simulink model "prob4_214869"  (R2020a)
settings: Solver=VariableStepAuto  StartTime=0.0  StopTime=10.0  RelTol=1e-3
settings Model: Creator=sonal  LastModifiedBy=sonal

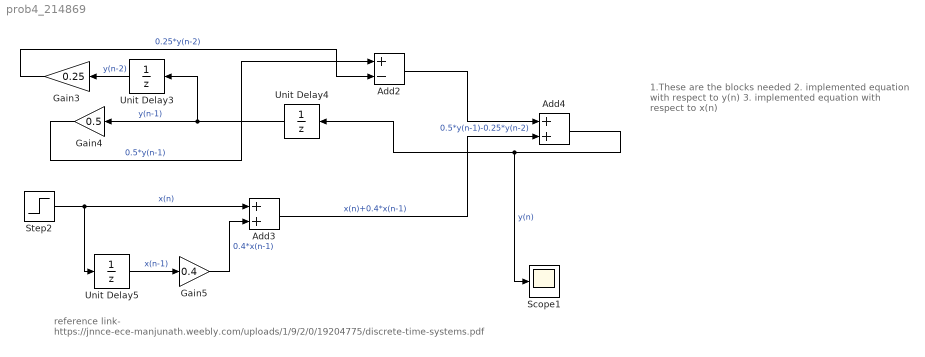
== system prob4_214869 ==
  note: reference link- https://jnnce-ece-manjunath.weebly.com/uploads/1/9/2/0/19204775/discrete-time-systems.pdf
  note: 1.These are the blocks needed
      | 2. implemented equation with respect to y(n)
      | 3. implemented equation with respect to x(n)
  Add2 : Sum  Inputs=+-
  Add3 : Sum
  Add4 : Sum
  Gain3 : Gain  Gain=0.25
  Gain4 : Gain  Gain=0.5
  Gain5 : Gain  Gain=0.4
  Scope1 : Scope
  Step2 : Step  SampleTime=0.01
  Unit Delay3 : UnitDelay  SampleTime=-1  HasFrameUpgradeWarning=on
  Unit Delay4 : UnitDelay  SampleTime=-1  HasFrameUpgradeWarning=on
  Unit Delay5 : UnitDelay  SampleTime=-1  HasFrameUpgradeWarning=on
  wires:
  Gain4/1 -> Add2/1  "0.5*y(n-1)"
  Gain3/1 -> Add2/2  "0.25*y(n-2)"
  Add4/1 -> Scope1/1, Unit Delay4/1  "y(n)"
  Unit Delay4/1 -> Unit Delay3/1, Gain4/1  "y(n-1)"
  Unit Delay3/1 -> Gain3/1  "y(n-2)"
  Step2/1 -> Unit Delay5/1, Add3/1  "x(n)"
  Gain5/1 -> Add3/2  "0.4*x(n-1)"
  Add3/1 -> Add4/2  "x(n)+0.4*x(n-1)"
  Unit Delay5/1 -> Gain5/1  "x(n-1)"
  Add2/1 -> Add4/1  "0.5*y(n-1)-0.25*y(n-2)"
